simulink model "Clevel_ROAD_ROUGHNESS"  (R2014a)
settings: Solver=ode45  StartTime=0.0  StopTime=10.0  RelTol=1e-3
libraries: simulink x1
settings Model: Creator=Administrator  LastModifiedBy=Administrator

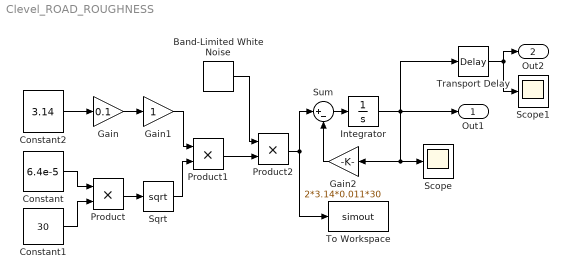
== system Clevel_ROAD_ROUGHNESS ==
  Band-Limited White Noise : simulink/Sources/Band-Limited White Noise  Cov=[0.1]  Ts=0.1  seed=[23341]
  Constant : Constant  Value=6.4e-5
  Constant1 : Constant  Value=30
  Constant2 : Constant  Value=3.14
  Gain : Gain  Gain=0.1
  Gain1 : Gain
  Gain2 : Gain  Gain=2*3.14*0.011*30
  Integrator : Integrator
  Product : Product
  Product1 : Product
  Product2 : Product
  Scope : Scope
  Scope1 : Scope
  Sqrt : Sqrt  SaturateOnIntegerOverflow=on
  Sum : Sum  Inputs=|+-
  To Workspace : ToWorkspace  VariableName=simout  SaveFormat=Structure With Time  SampleTime=-1
  Transport Delay : TransportDelay
  Out1 : Outport
  Out2 : Outport  Port=2
  wires:
  Constant/1 -> Product/1
  Constant1/1 -> Product/2
  Product/1 -> Sqrt/1
  Constant2/1 -> Gain/1
  Gain/1 -> Gain1/1
  Gain1/1 -> Product1/1
  Sqrt/1 -> Product1/2
  Band-Limited White Noise/1 -> Product2/1
  Product1/1 -> Product2/2
  Transport Delay/1 -> Scope1/1, Out2/1
  Product2/1 -> Sum/1, To Workspace/1
  Sum/1 -> Integrator/1
  Integrator/1 -> Gain2/1, Scope/1, Out1/1, Transport Delay/1
  Gain2/1 -> Sum/2
